simulink model "simulink_validacao"  (R2016a)
settings: Solver=VariableStepAuto  StartTime=0.0  StopTime=10.0  RelTol=1e-3
values from neighbouring files (symbols this model uses):
  f_mol_ar = [0.79 0.21 0.0 0 0 0 0 0]    [codigo_validacao.m]
  f_mol_gas = [0.76 0 0 0 0.11 0.13 0 0]    [codigo_validacao.m]
  m_c = 0.3    [codigo_validacao.m]
  m_f = 0.01    [codigo_validacao.m]
  N = 0.82    [codigo_validacao.m]
  Pc_i = 368000    [codigo_validacao.m]
  Ph_i = 105000    [codigo_validacao.m]
  Tc_i = 358.15    [codigo_validacao.m]
  Th_i = 584.817    [codigo_validacao.m]
(part 3 of 4)

== matlab function simulink_validacao/Recuperdor de calor CWPS/Densidade Fluido Frio/densidade_c_ch ==
  data: t input; y output; p input; frac_mol input
function y = rho(t,p,frac_mol)
%#codegen
%
%------------------- FUNÇÃO DENSIDADE DOS GASES -------------------------
%
%   -Autor: Janderson Honório Mazzine Afonso
%   -Email: janderson.mazzine2015@engenharia.ufjf.br
%   -Ano: 2020
%   -Referência: IUPAC. Periodic Table of Elements. Disponivel em
%   <https://iupac.org/what-we-do/periodic-table-of-elements/> Acesso em
%   01 set. 2020.
%   -Citar como: AFONSO. Janderson H. M. Densidade dos Gases de Combustão
%                Aplicados em Turbinas a Gás. UFJF, 2020.
%   -Versão: 01.09.2020
%
%----------------------- DESCRIÇÃO DA FUNÇÃO ------------------------------
%
%   A presente função retorna a densidade, em [kg/m^3] de um gás puro ou 
%   mistura de gases ideais segundo a equação de Clapeyron, considerando as
%   massas molares dos atomos na tabela da IUPAC
%
%--------------------------- INSTRUÇÕES -----------------------------------
%
%              [rho] = densi_gas( t, p, frac_mol)
%
%   A temperatura de entrada deve ser dada em Kelvin [K], a pressão em mega
%   Pascal [Pa]. As frações molares devem ser dada em um vetor com o  
%   seguinte formato:
%
%                 (%N2 %O2 %Ar %Ne %H2O %CO2 %CO %SO2)
%
%   Caso alguma das espécies não faça parte da mistura deve ser atribuido o
%   valor 0 (zero) a sua posição no vetor. A soma das frações de cada espé-
%   cie deve ser sempre igual a 1.
%
%------------------------ MENSAGEM DE ERRO -------------------------------- 
%
%   Uma mensagem de erro será exibida caso a soma das concentrações dos 
%   componentes do gás em estudo seja diferente de 1.
%
%---------------------------- EXEMPLOS ------------------------------------
%
%   1)Definir a densidade do ar atmosférico considerando uma composição de 
%   Oxigênio (21%) e Nitrogênio (79%) apenas, a 100ºC e 2 atm.
%
%   t = 373.15;
%   p = 0.202650;
%   frac_mol = [0.79 0.21 0 0 0 0 0 0];
%   [rho] = densi_gas( t, p, frac_mol);
%
%   ANS: 1.88444931513629e+000
%   
%--------------------------------------------------------------------------

if  sum(frac_mol) ~= 1 %checa composição informada
    error('A soma das frações de composição é diferente de 1')
end

mm_el = [28.014 31.998 39.95 20.180 33.006 44.009 28.01 64.058]; %massa molar dos gases puros segundo IUPAC 2020, [g/mol]

rho = 0; 
R=8.314462; %Constante dos gases, em [m^3 Pa kg^-1 mol^-1]
    for j = 1:8, %percorre espécies
        if frac_mol(j) > 0  %evita o cálculo das especies com concentração nula
            rho=rho+(((mm_el(j)*10^(-3))*frac_mol(j)*(p))/(R*t)); 
        end
    end
    
    y = rho;

== matlab function simulink_validacao/Recuperdor de calor CWPS/Troca de Calor/Condutividade/cond_c_ch ==
  data: t input; y output; frac_mol input
function y = k(t, frac_mol)
%#codegen
%
%------------------ FUNÇÃO CONDUTIVIDADE DOS GASES ------------------------
%
%   -Autor: Janderson Honório Mazzine Afonso
%   -Email: janderson.mazzine2015@engenharia.ufjf.br
%   -Ano: 2020
%
%   -Referências: 
%   [1]MATOS, M. A. A. Propriedades termofísicas de algunsgases, sólidos e  
%   da água. Aveiro: Editora da Universidade de Aveiro, 1998.
%   [2]BIRD R. B., WARREN E. S., and EDWIN N. L. Transport Phenomena. 2nd 
%   ed. New York: Jonh Wiley & Sons, 2002.
%   [3]IUPAC. Periodic Table of Elements. Disponivel em
%   <https://iupac.org/what-we-do/periodic-table-of-elements/> Acesso em
%   01 set. 2020.
%
%   -Citar como: AFONSO. Janderson H. M. Condutividade dos Gases de 
%                Combustão Aplicados em Turbinas a Gás. UFJF, 2020.
%   -Versão: 03.09.2020
%
%----------------------- DESCRIÇÃO DA FUNÇÃO ------------------------------
%
%   A presente função retorna a condutividade, em [W/m.K] de um gás puro 
%   segundo a expressão e coeficientes de regressão apresentados por Matos  
%   [1], e da mistura considerando também a correlação semiempírica 
%   desenvolvida por Wilke e apresentada no livro de Bird [2], considerando
%   as massas molares dos atomos na tabela da IUPAC [3].
%
%--------------------------- INSTRUÇÕES -----------------------------------
%
%                   [k] = cond_gas( t, frac_mol)
%
%   A temperatura de entrada deve ser dada em Kelvin [K] e as frações 
%   molares devem ser dada em um vetor com o seguinte formato:
%   
%                 (%N2 %O2 %Ar %Ne %H2O %CO2 %CO %SO2)
%
%   Caso alguma das espécies não faça parte da mistura deve ser atribuido o
%   valor 0 (zero) a sua posição no vetor. A soma das frações de cada espé-
%   cie deve ser sempre igual a 1.
%   
%   Porém, o presente modelo não contempla o gas neônio. Caso seja
%   necessário, deve-se implementar seus coeficientes na matriz.
%
%-------------------- MENSAGEM DE ERRO E AVISOS --------------------------- 
%
%   Uma mensagem de erro será exibida caso a soma das concentrações dos 
%   componentes do gás em estudo seja diferente de 1, ou caso tente-se 
%   computar um gás que possua Neônio em sua composição, o qual não é 
%   contemplado no presente modelo.
%   
%   Um aviso será exibido caso a temperatura desejada da mistura esteja
%   fora do intervalo de temperatura de algum dos gases puros que a compõe,
%   conforme a tabela abaixo:
%
%              Gas	|	T_min (K)	|	T_max (K)
%               ---------------------------------
%               N2 		  250 			  1500
%               O2		  250 			  1500
%               Ar		  110			  1300
%               Ne		  NaN			  NaN
%               H2O 	  400 			  1500
%               CO2 	  250 			  1500 
%               CO		  250 			  1500
%               SO2 	  170 			  1700
%
%---------------------------- EXEMPLOS ------------------------------------
%
%   1)Definir a condutividade do ar atmosférico considerando uma composição 
%   de Oxigênio (21%) e Nitrogênio (79%) apenas, a 100ºC.
%
%   t = 373.15;
%   f_mol = [0.79 0.21 0 0 0 0 0 0];
%   [k] = cond_gas( t, f_mol)
%
%   ANS: 30.8821778098117e-003
%   
%--------------------------------------------------------------------------


if  sum(frac_mol) ~= 1 %checa composição informada
    error('A soma das frações de composição é diferente de 1');
elseif frac_mol(4) ~= 0
    error('Erro: Gás Neonio não contemplado no modelo');
end

mm_el = [28.014 31.998 39.95 20.180 33.006 44.009 28.01 64.058]; %massa molar dos gases puros segundo IUPAC 2020, [g/mol]

k = 0;
cont = 0;
cond = zeros(1, 8);
vis = zeros(1, 8);
fm = zeros(1, 8);
mm = zeros(1, 8);
psi_ab = zeros(1, 8);

coef_cond = [0.47088*10^(-2)	0.78562*10^(-4) 	-0.26266*10^(-7) 	0.55540*10^(-11) 	250 	1500;
            0.33470*10^(-2) 	0.81930*10^(-4) 	-0.16987*10^(-7) 	0.29881*10^(-11) 	250 	1500;
            0.27132*10^(-2) 	0.55394*10^(-4) 	-0.21772*10^(-7) 	0.55268*10^(-11) 	110 	1500;
            0                   0                   0                   0                   0       0;
            -0.79293*10^(-2) 	0.76030*10^(-4) 	0.31270*10^(-7) 	-0.10805*10^(-10)	400 	1500;
            -0.95947*10^(-2) 	0.92700*10^(-4) 	-0.19366*10^(-7) 	0.32189*10^(-11) 	250 	1500;
            0.10224*10^(-2)		0.89079*10^(-4) 	-0.32557*10^(-7) 	0.89390*10^(-11) 	250 	1500;
            -0.80851*10^(-2)	0.63433*10^(-4) 	-0.13817*10^(-7) 	0.23028*10^(-11) 	300     1700];


coef_visc = [0.31619*10^(-5)	0.56192*10^(-7) 	-0.24148*10^(-10)  	0.61370*10^(-14) 	250 	1500;
            0.26918*10^(-5)		0.68519*10^(-7)  	-0.29857*10^(-10) 	0.75600*10^(-14) 	250 	1500;
            0.50458*10^(-5)		0.63459*10^(-7)  	-0.17506*10^(-10) 	0.37009*10^(-14) 	250     1300;
            0                   0                   0                   0                   0       0;
            -0.41991*10^(-5) 	0.45336E-07    		-0.50749*10^(-11) 	0.15526*10^(-14) 	400 	1500;
            -0.16636*10^(-5)	0.63064*10^(-7)  	-0.26223*10^(-10) 	0.58813*10^(-14) 	250 	1500; 
            0.30012*10^(-5)		0.56504*10^(-7)  	-0.23998*10^(-10) 	0.62734*10^(-14) 	250 	1500; 
            0-.37930*10^(-5)	0.46450*10^(-7) 	-0.72760*10^(-11) 	0                   170 	1700];

    for i = 1:8, %percorre espécies
        if frac_mol(i) ~= 0  %evita o cálculo das especies com concentração nula
            cont=cont+1;
            fm(cont)= frac_mol(i);
            mm(cont)= mm_el(i);
            vis(cont)=coef_visc(i,1)+coef_visc(i,2)*t+coef_visc(i,3)*t^2+coef_visc(i,4)*t^3;
            cond(cont)=coef_cond(i,1)+coef_cond(i,2)*t+coef_cond(i,3)*t^2+coef_cond(i,4)*t^3;
            if t<coef_visc(i,5)||t<coef_cond(i,5)
                error('A temperatura está abaixo do limite de aplicabilidade do modelo para o gas abaixo:')
                %disp(n_esp(i));
            elseif t>coef_visc(i,6)||t>coef_cond(i,6)
                error('A temperatura está acima do limite de aplicabilidade do modelo para os gas abaixo:')
                %disp(n_esp(i));
            end
        end
    end
    
    for a = 1:cont, %calculo psi
        for b = 1:cont,
            psi_ab(a)=psi_ab(a)+fm(b)*((1/sqrt(8))*(1+mm(a)/mm(b))^(-0.5)*(1+(vis(a)/vis(b))^(0.5)*(mm(b)/mm(a))^(0.25))^2);
        end
        k=k+((fm(a)*cond(a))/psi_ab(a));
    end    
y = k;

== matlab function simulink_validacao/Recuperdor de calor CWPS/Calculos Exergéticos Enstropia e Entalpia/h_c_i ==
  data: t input; y output; frac_mol input
function y = entalpia(t, frac_mol)
%#codegen
%
%------------------- FUNÇÃO ENTALPIA DOS GASES -------------------------
%
%   -Autor: Janderson Honório Mazzine Afonso
%   -Email: janderson.mazzine2015@engenharia.ufjf.br
%   -Ano: 2020
%   -Referência: BUCKER, D.; SPAN, R.; WAGNER, W. Thermodynamic property 
%                models for moist air and combustion gases. J. Eng. Gas 
%                Turbines Power, v. 125, n. 1, p. 374-384, 2003.
%                https://doi.org/10.1115/1.1520154
%   -Citar como: AFONSO. Janderson H. M. Propriedade dos Gases de Combustão
%                Aplicados em Turbinas a Gás - Entalpia. UFJF, 2020.
%   -Versão: 14.05.2020
%
%----------------------- DESCRIÇÃO DA FUNÇÃO ------------------------------
%
%   A presente função retorna a entalpia em J/K de uma mistura de gases que
%   compõe o ar e produtos da combustão para temperaturas entre 200 e 3300 
%   Kelvin de acordo com o modelo proposto por BUCKER, SPAN e WAGNER (2003)
%   em seu trabalho "Thermodynamic Property Model for Moist Air and Combus-
%   tion Gases" a partir da temperatura da mistura e sua composição molar.
%
%--------------------------- INSTRUÇÕES -----------------------------------
%
%                       [h] = entalpia( t, frac_mol)
%
%   A temperatura de entrada deve ser dada em Kelvin [K] e a composição 
%   molar da mistura em fração molar dos componentes. As frações molares 
%   devem ser dada em um vetor com o seguinte formato:
%
%                 (%N2 %O2 %Ar %Ne %H2O %CO2 %CO %SO2)
%
%   Caso alguma das espécies não faça parte da mistura deve ser atribuido o
%   valor 0 (zero) a sua posição no vetor. A soma das frações de cada espé-
%   cie deve ser sempre igual a 1.
%
%----------------------------- ATENÇÃO ------------------------------------ 
%
%   Recomenda-se a adoção deste código para o calculo da variação da
%   entalpia entre dois pontos do fluido, e não para o calculo de um ponto
%   isolado. Distorções nos valores de diferentes modelos propostos podem
%   ser observadas devido as condições de referência, porém a variação da
%   entropia entre dois posntos (estados)deverá ser equivalente mesmo em
%   modelos distintos.
%
%------------------------ MENSAGEM DE ERRO -------------------------------- 
%
%   Uma mensagem de erro será exibida caso a temperatura
%   informada esteja fora dos limites de validade do modelo (entre 200 e
%   3300 K) ou caso a soma das concentrações dos componentes do gás em
%   estudo seja diferente de 1.
%
%---------------------------- EXEMPLOS ------------------------------------
%
%   1)Definir a entalpia em J/K do ar atmosférico considerando uma composi-
%   ção de Oxigênio (21%) e Nitrogênio (79%) apenas, a 30ºC.    
%
%   t = 303.15;
%   f_mol = [0.79 0.21 0 0 0 0 0 0]
%   [h] = entalpia( t, f_mol )
%
%   ANS:
%   h = 30.4129989891052e+003
%
%--------------------------------------------------------------------------


if t < 200 || t > 3300 %checa aplicabilidade do modelo
    error('Temperatura informada fora do intervalo de validade do modelo(200 K < T < 3300 K)')
elseif sum(frac_mol) ~= 1 %checa composição informada
    error('A soma das frações de composição é diferente de 1')
end

b_i = [0.00 -1.50 -1.25 -0.75 -0.50 -0.25 0.25 0.50 0.75 1.00];
%b_i : vetor de coeficientes bi

a_k = [4.305300363*10^8 -4.085709350*10^6 ;
       5.295253592*10^7 -7.353805669*10^5 ;
       -5.677745067*10^3 0 ;
       -5.677745067*10^3 0 ;
       -7.574888563*10^8 7.373724814*10^6 ;
       2.042361458*10^8 -1.912121053*10^6 ;
       4.306836224*10^8 -4.203685809*10^6 ;
       -3.845730250*10^8 3.543224735*10^6]; 
%a_k : matriz coef. ak_I e ak_II (colunas) e especies (linhas)
   
a_ki = [2.475830346*10^6 -2.815239891*10^4 1.116401165*10^5 -8.147644187*10^5 2.185120405*10^6 -2.978031305*10^6 -1.308008001*10^6 4.305948510*10^5 -8.082302563*10^4 6.622545214*10^3;
        6.408242565*10^5 -1.599937045*10^3 9.984801256*10^3 -1.280873444*10^5 4.186599156*10^5 -6.720142804*10^5 -3.799977202*10^5 1.378691801*10^5 -2.806954185*10^4 2.459943097*10^3;
        2.078618000*10^1 0 0 0 0 0 0 0 0 0; 
        2.078618000*10^1 0 0 0 0 0 0 0 0 0;
        -4.747782033*10^6 4.799919289*10^4 -1.931588954*10^5 1.460728340*10^6 -4.000075762*10^6 5.576209858*10^6 2.570488297*10^6 -8.670521019*10^5 1.666429390*10^5 -1.396634620*10^4;
        1.103695150*10^6 -1.365096910*10^4 5.357704944*10^4 -3.816063864*10^5 1.008950325*10^6 -1.352938737*10^6 -5.701809626*10^5 1.828513133*10^5 -3.329618224*10^4 2.635366727*10^3;
        2.670755728*10^6 -2.715629936*10^4 1.096509012*10^5 -8.303525865*10^5 2.269213594*10^6 -3.151865706*10^6 -1.438126165*10^6 4.824833432*10^5 -9.227524508*10^4 7.701550175*10^3;
        -2.076653674*10^6 2.589571253*10^4 -1.012523438*10^5 7.161863952*10^5 -1.889754780*10^6 2.535020356*10^6 1.082842148*10^6 -3.524395911*10^5 6.552035769*10^4 -5.325634796*10^3;]; 
%a_ki : matriz coef. ak_i, i = (1:10) (colunas) e especies (linhas)

t_0 = 273.15; %Temperatura de referência, em K

a_mix_gr=[0 0];
a_mix_i=[0 0 0 0 0 0 0 0 0 0];
mm_esp = [28.014 31.998 39.963 20.180 18.015 40.019 28.009 64.063];
mm_mis=0;

for i = 1:8, %Percorre espécies
          if frac_mol(i) > 0  %evita o cálculo das especies com concentração nula
              a_mix_gr(1)=a_mix_gr(1)+a_k(i,1)*frac_mol(i)*(1000/mm_esp(i));
              a_mix_gr(2)=a_mix_gr(2)+a_k(i,2)*frac_mol(i)*(1000/mm_esp(i));
              sum_delta_s0=frac_mol(i)*log(frac_mol(i))*(1000/mm_esp(i));
              mm_mis= mm_mis+frac_mol(i)/(1000/mm_esp(i));

              for j = 1:10, %percorre coeficientes
                  a_mix_i(j)=a_mix_i(j)+a_ki(i,j)*frac_mol(i)*(1000/mm_esp(i));
              end
          end
end

%Calculo entalpia
sum_h0=0;

for i = 1:10,  
    
    sum_h0=sum_h0+a_mix_i(i)*(t_0/(b_i(i)+1))*((t/t_0)^(b_i(i)+1));
            
end              
          
  h= a_mix_gr(1)+sum_h0;
  y = h;

== matlab function simulink_validacao/Recuperdor de calor CWPS/Calculos Exergéticos Enstropia e Entalpia/s_c_i ==
  data: t input; p input; y output; frac_mol input
function y = entropia(t, p, frac_mol)
%#codegen
%
%--------------------- FUNÇÃO ENTROPIA DOS GASES --------------------------
%
%   -Autor: Janderson Honório Mazzine Afonso
%   -Email: janderson.mazzine2015@engenharia.ufjf.br
%   -Ano: 2020
%   -Referência: BUCKER, D.; SPAN, R.; WAGNER, W. Thermodynamic property 
%                models for moist air and combustion gases. J. Eng. Gas 
%                Turbines Power, v. 125, n. 1, p. 374-384, 2003.
%                https://doi.org/10.1115/1.1520154
%   -Citar como: AFONSO. Janderson H. M. Propriedade dos Gases de Combustão
%                Aplicados em Turbinas a Gás - Entropia. UFJF, 2020.
%   -Versão: 14.05.2020
%
%----------------------- DESCRIÇÃO DA FUNÇÃO ------------------------------
%
%   A presente função retorna a entropia em J/kg.K de uma mistura de gases  
%   que compõe o ar e produtos da combustão para temperaturas entre 200 e 
%   3300 Kelvin de acordo com o modelo proposto por BUCKER, SPAN e WAGNER 
%   (2003) em seu trabalho "Thermodynamic Property Model for Moist Air and
%   Combustion Gases" a partir da temperatura da mistura e sua composição
%   molar.
%
%--------------------------- INSTRUÇÕES -----------------------------------
%
%                       [s] = s( t, p, frac_mol)
%
%   A temperatura de entrada deve ser dada em Kelvin [K], a pressão em Pas-
%   cal [Pa] e a composição molar da mistura em fração molar dos componen-
%   tes. As frações molares devem ser dada em um vetor com o seguinte for-
%   mato:
%
%                 (%N2 %O2 %Ar %Ne %H2O %CO2 %CO %SO2)
%
%   Caso alguma das espécies não faça parte da mistura deve ser atribuido o
%   valor 0 (zero) a sua posição no vetor. A soma das frações de cada espé-
%   cie deve ser sempre igual a 1.
%
%----------------------------- ATENÇÃO ------------------------------------ 
%
%   Recomenda-se a adoção deste código para o calculo da variação da
%   entropia entre dois pontos do fluido, e não para o calculo de um ponto
%   isolado. Distorções nos valores de diferentes modelos propostos podem
%   ser observadas devido as condições de referência, porém a variação da
%   entropia entre dois posntos (estados)deverá ser equivalente mesmo em
%   modelos distintos.
%
%------------------------ MENSAGEM DE ERRO -------------------------------- 
%
%   Uma mensagem de erro será exibida caso a temperatura informada esteja
%   fora dos limites de validade do modelo (entre 200 e 3300 K) ou caso a 
%   soma das concentrações dos componentes do gás em estudo seja diferente
%   de 1.
%
%---------------------------- EXEMPLOS ------------------------------------
%
%   1)Definir a entropia do ar atmosférico em J/kg.K considerando uma com- 
%   posição de Oxigênio (21%) e Nitrogênio (79%) apenas, a 30ºC e a 1 atm.
%
%   t = 303.15;
%   p = 101325;
%   f_mol = [0.79 0.21 0 0 0 0 0 0]
%   [s] = entropia( t, p, f_mol )
%
%   ANS:
%   s = 190.795467689633e+000
%
%--------------------------------------------------------------------------

if t < 200 || t > 3300 %checa aplicabilidade do modelo
    error('Temperatura informada fora do intervalo de validade do modelo(200 K < T < 3300 K)')
elseif sum(frac_mol) ~= 1 %checa composição informada
    error('A soma das frações de composição é diferente de 1')
end


b_i = [0.00 -1.50 -1.25 -0.75 -0.50 -0.25 0.25 0.50 0.75 1.00];
%b_i : vetor de coeficientes bi

a_k = [4.305300363*10^8 -4.085709350*10^6 ;
       5.295253592*10^7 -7.353805669*10^5 ;
       -5.677745067*10^3 0 ;
       -5.677745067*10^3 0 ;
       -7.574888563*10^8 7.373724814*10^6 ;
       2.042361458*10^8 -1.912121053*10^6 ;
       4.306836224*10^8 -4.203685809*10^6 ;
       -3.845730250*10^8 3.543224735*10^6]; 
%a_k : matriz coef. ak_I e ak_II (colunas) e especies (linhas)
   
a_ki = [2.475830346*10^6 -2.815239891*10^4 1.116401165*10^5 -8.147644187*10^5 2.185120405*10^6 -2.978031305*10^6 -1.308008001*10^6 4.305948510*10^5 -8.082302563*10^4 6.622545214*10^3;
        6.408242565*10^5 -1.599937045*10^3 9.984801256*10^3 -1.280873444*10^5 4.186599156*10^5 -6.720142804*10^5 -3.799977202*10^5 1.378691801*10^5 -2.806954185*10^4 2.459943097*10^3;
        2.078618000*10^1 0 0 0 0 0 0 0 0 0; 
        2.078618000*10^1 0 0 0 0 0 0 0 0 0;
        -4.747782033*10^6 4.799919289*10^4 -1.931588954*10^5 1.460728340*10^6 -4.000075762*10^6 5.576209858*10^6 2.570488297*10^6 -8.670521019*10^5 1.666429390*10^5 -1.396634620*10^4;
        1.103695150*10^6 -1.365096910*10^4 5.357704944*10^4 -3.816063864*10^5 1.008950325*10^6 -1.352938737*10^6 -5.701809626*10^5 1.828513133*10^5 -3.329618224*10^4 2.635366727*10^3;
        2.670755728*10^6 -2.715629936*10^4 1.096509012*10^5 -8.303525865*10^5 2.269213594*10^6 -3.151865706*10^6 -1.438126165*10^6 4.824833432*10^5 -9.227524508*10^4 7.701550175*10^3;
        -2.076653674*10^6 2.589571253*10^4 -1.012523438*10^5 7.161863952*10^5 -1.889754780*10^6 2.535020356*10^6 1.082842148*10^6 -3.524395911*10^5 6.552035769*10^4 -5.325634796*10^3;]; 
%a_ki : matriz coef. ak_i, i = (1:10) (colunas) e especies (linhas)

t_0 = 273.15; %Temperatura de referência, em K
p_0 = 0.101325; %Pressão de referência, em MPa
r_m = 8.314472; %Constante dos gases, em J/(mol*K)
p=p/10^6; %converte Pa na entrada para MPa para os cálculos do modelo

a_mix_gr=[0 0];
a_mix_i=[0 0 0 0 0 0 0 0 0 0];
mm_esp = [28.014 31.998 39.963 20.180 18.015 40.019 28.009 64.063];
mm_mis=0;
sum_delta_s0=0;

for i = 1:8, %Percorre espécies
          if frac_mol(i) > 0  %evita o cálculo das especies com concentração nula
              a_mix_gr(1)=a_mix_gr(1)+a_k(i,1)*frac_mol(i)*(1000/mm_esp(i));
              a_mix_gr(2)=a_mix_gr(2)+a_k(i,2)*frac_mol(i)*(1000/mm_esp(i));
              sum_delta_s0=frac_mol(i)*log(frac_mol(i))*(1000/mm_esp(i));
              mm_mis= mm_mis+frac_mol(i)/(1000/mm_esp(i));

              for j = 1:10, %percorre coeficientes
                  a_mix_i(j)=a_mix_i(j)+a_ki(i,j)*frac_mol(i)*(1000/mm_esp(i));
              end
          end
end

delta_s0=(-r_m)*sum_delta_s0;

%Calculo entropia

sum_s0=0;
r = r_m/mm_mis; %Constante particular do gas, em J/(kg*K)

for i = 2:10,  
    
    sum_s0=sum_s0+(a_mix_i(i)/b_i(i))*((t/t_0)^b_i(i));
            
end          
          
s=a_mix_gr(2)-(r*log(p/p_0))+delta_s0+(a_mix_i(1)*log(t/t_0))+sum_s0;

  y = s;

== matlab function simulink_validacao/Recuperdor de calor CWPS/Calculos Exergéticos Enstropia e Entalpia/h_c_o ==
  data: t input; y output; frac_mol input
function y = entalpia(t, frac_mol)
%#codegen
%
%------------------- FUNÇÃO ENTALPIA DOS GASES -------------------------
%
%   -Autor: Janderson Honório Mazzine Afonso
%   -Email: janderson.mazzine2015@engenharia.ufjf.br
%   -Ano: 2020
%   -Referência: BUCKER, D.; SPAN, R.; WAGNER, W. Thermodynamic property 
%                models for moist air and combustion gases. J. Eng. Gas 
%                Turbines Power, v. 125, n. 1, p. 374-384, 2003.
%                https://doi.org/10.1115/1.1520154
%   -Citar como: AFONSO. Janderson H. M. Propriedade dos Gases de Combustão
%                Aplicados em Turbinas a Gás - Entalpia. UFJF, 2020.
%   -Versão: 14.05.2020
%
%----------------------- DESCRIÇÃO DA FUNÇÃO ------------------------------
%
%   A presente função retorna a entalpia em J/K de uma mistura de gases que
%   compõe o ar e produtos da combustão para temperaturas entre 200 e 3300 
%   Kelvin de acordo com o modelo proposto por BUCKER, SPAN e WAGNER (2003)
%   em seu trabalho "Thermodynamic Property Model for Moist Air and Combus-
%   tion Gases" a partir da temperatura da mistura e sua composição molar.
%
%--------------------------- INSTRUÇÕES -----------------------------------
%
%                       [h] = entalpia( t, frac_mol)
%
%   A temperatura de entrada deve ser dada em Kelvin [K] e a composição 
%   molar da mistura em fração molar dos componentes. As frações molares 
%   devem ser dada em um vetor com o seguinte formato:
%
%                 (%N2 %O2 %Ar %Ne %H2O %CO2 %CO %SO2)
%
%   Caso alguma das espécies não faça parte da mistura deve ser atribuido o
%   valor 0 (zero) a sua posição no vetor. A soma das frações de cada espé-
%   cie deve ser sempre igual a 1.
%
%----------------------------- ATENÇÃO ------------------------------------ 
%
%   Recomenda-se a adoção deste código para o calculo da variação da
%   entalpia entre dois pontos do fluido, e não para o calculo de um ponto
%   isolado. Distorções nos valores de diferentes modelos propostos podem
%   ser observadas devido as condições de referência, porém a variação da
%   entropia entre dois posntos (estados)deverá ser equivalente mesmo em
%   modelos distintos.
%
%------------------------ MENSAGEM DE ERRO -------------------------------- 
%
%   Uma mensagem de erro será exibida caso a temperatura
%   informada esteja fora dos limites de validade do modelo (entre 200 e
%   3300 K) ou caso a soma das concentrações dos componentes do gás em
%   estudo seja diferente de 1.
%
%---------------------------- EXEMPLOS ------------------------------------
%
%   1)Definir a entalpia em J/K do ar atmosférico considerando uma composi-
%   ção de Oxigênio (21%) e Nitrogênio (79%) apenas, a 30ºC.    
%
%   t = 303.15;
%   f_mol = [0.79 0.21 0 0 0 0 0 0]
%   [h] = entalpia( t, f_mol )
%
%   ANS:
%   h = 30.4129989891052e+003
%
%--------------------------------------------------------------------------


if t < 200 || t > 3300 %checa aplicabilidade do modelo
    error('Temperatura informada fora do intervalo de validade do modelo(200 K < T < 3300 K)')
elseif sum(frac_mol) ~= 1 %checa composição informada
    error('A soma das frações de composição é diferente de 1')
end

b_i = [0.00 -1.50 -1.25 -0.75 -0.50 -0.25 0.25 0.50 0.75 1.00];
%b_i : vetor de coeficientes bi

a_k = [4.305300363*10^8 -4.085709350*10^6 ;
       5.295253592*10^7 -7.353805669*10^5 ;
       -5.677745067*10^3 0 ;
       -5.677745067*10^3 0 ;
       -7.574888563*10^8 7.373724814*10^6 ;
       2.042361458*10^8 -1.912121053*10^6 ;
       4.306836224*10^8 -4.203685809*10^6 ;
       -3.845730250*10^8 3.543224735*10^6]; 
%a_k : matriz coef. ak_I e ak_II (colunas) e especies (linhas)
   
a_ki = [2.475830346*10^6 -2.815239891*10^4 1.116401165*10^5 -8.147644187*10^5 2.185120405*10^6 -2.978031305*10^6 -1.308008001*10^6 4.305948510*10^5 -8.082302563*10^4 6.622545214*10^3;
        6.408242565*10^5 -1.599937045*10^3 9.984801256*10^3 -1.280873444*10^5 4.186599156*10^5 -6.720142804*10^5 -3.799977202*10^5 1.378691801*10^5 -2.806954185*10^4 2.459943097*10^3;
        2.078618000*10^1 0 0 0 0 0 0 0 0 0; 
        2.078618000*10^1 0 0 0 0 0 0 0 0 0;
        -4.747782033*10^6 4.799919289*10^4 -1.931588954*10^5 1.460728340*10^6 -4.000075762*10^6 5.576209858*10^6 2.570488297*10^6 -8.670521019*10^5 1.666429390*10^5 -1.396634620*10^4;
        1.103695150*10^6 -1.365096910*10^4 5.357704944*10^4 -3.816063864*10^5 1.008950325*10^6 -1.352938737*10^6 -5.701809626*10^5 1.828513133*10^5 -3.329618224*10^4 2.635366727*10^3;
        2.670755728*10^6 -2.715629936*10^4 1.096509012*10^5 -8.303525865*10^5 2.269213594*10^6 -3.151865706*10^6 -1.438126165*10^6 4.824833432*10^5 -9.227524508*10^4 7.701550175*10^3;
        -2.076653674*10^6 2.589571253*10^4 -1.012523438*10^5 7.161863952*10^5 -1.889754780*10^6 2.535020356*10^6 1.082842148*10^6 -3.524395911*10^5 6.552035769*10^4 -5.325634796*10^3;]; 
%a_ki : matriz coef. ak_i, i = (1:10) (colunas) e especies (linhas)

t_0 = 273.15; %Temperatura de referência, em K

a_mix_gr=[0 0];
a_mix_i=[0 0 0 0 0 0 0 0 0 0];
mm_esp = [28.014 31.998 39.963 20.180 18.015 40.019 28.009 64.063];
mm_mis=0;

for i = 1:8, %Percorre espécies
          if frac_mol(i) > 0  %evita o cálculo das especies com concentração nula
              a_mix_gr(1)=a_mix_gr(1)+a_k(i,1)*frac_mol(i)*(1000/mm_esp(i));
              a_mix_gr(2)=a_mix_gr(2)+a_k(i,2)*frac_mol(i)*(1000/mm_esp(i));
              sum_delta_s0=frac_mol(i)*log(frac_mol(i))*(1000/mm_esp(i));
              mm_mis= mm_mis+frac_mol(i)/(1000/mm_esp(i));

              for j = 1:10, %percorre coeficientes
                  a_mix_i(j)=a_mix_i(j)+a_ki(i,j)*frac_mol(i)*(1000/mm_esp(i));
              end
          end
end

%Calculo entalpia
sum_h0=0;

for i = 1:10,  
    
    sum_h0=sum_h0+a_mix_i(i)*(t_0/(b_i(i)+1))*((t/t_0)^(b_i(i)+1));
            
end              
          
  h= a_mix_gr(1)+sum_h0;
  y = h;

== matlab function simulink_validacao/Recuperdor de calor CWPS/Densidade Fluido Quente/densidade_h_i ==
  data: t input; y output; p input; frac_mol input
function y = rho(t,p,frac_mol)
%#codegen
%
%------------------- FUNÇÃO DENSIDADE DOS GASES -------------------------
%
%   -Autor: Janderson Honório Mazzine Afonso
%   -Email: janderson.mazzine2015@engenharia.ufjf.br
%   -Ano: 2020
%   -Referência: IUPAC. Periodic Table of Elements. Disponivel em
%   <https://iupac.org/what-we-do/periodic-table-of-elements/> Acesso em
%   01 set. 2020.
%   -Citar como: AFONSO. Janderson H. M. Densidade dos Gases de Combustão
%                Aplicados em Turbinas a Gás. UFJF, 2020.
%   -Versão: 01.09.2020
%
%----------------------- DESCRIÇÃO DA FUNÇÃO ------------------------------
%
%   A presente função retorna a densidade, em [kg/m^3] de um gás puro ou 
%   mistura de gases ideais segundo a equação de Clapeyron, considerando as
%   massas molares dos atomos na tabela da IUPAC
%
%--------------------------- INSTRUÇÕES -----------------------------------
%
%              [rho] = densi_gas( t, p, frac_mol)
%
%   A temperatura de entrada deve ser dada em Kelvin [K], a pressão em mega
%   Pascal [Pa]. As frações molares devem ser dada em um vetor com o  
%   seguinte formato:
%
%                 (%N2 %O2 %Ar %Ne %H2O %CO2 %CO %SO2)
%
%   Caso alguma das espécies não faça parte da mistura deve ser atribuido o
%   valor 0 (zero) a sua posição no vetor. A soma das frações de cada espé-
%   cie deve ser sempre igual a 1.
%
%------------------------ MENSAGEM DE ERRO -------------------------------- 
%
%   Uma mensagem de erro será exibida caso a soma das concentrações dos 
%   componentes do gás em estudo seja diferente de 1.
%
%---------------------------- EXEMPLOS ------------------------------------
%
%   1)Definir a densidade do ar atmosférico considerando uma composição de 
%   Oxigênio (21%) e Nitrogênio (79%) apenas, a 100ºC e 2 atm.
%
%   t = 373.15;
%   p = 0.202650;
%   frac_mol = [0.79 0.21 0 0 0 0 0 0];
%   [rho] = densi_gas( t, p, frac_mol);
%
%   ANS: 1.88444931513629e+000
%   
%--------------------------------------------------------------------------

if  sum(frac_mol) ~= 1 %checa composição informada
    error('A soma das frações de composição é diferente de 1')
end

mm_el = [28.014 31.998 39.95 20.180 33.006 44.009 28.01 64.058]; %massa molar dos gases puros segundo IUPAC 2020, [g/mol]

rho = 0; 
R=8.314462; %Constante dos gases, em [m^3 Pa kg^-1 mol^-1]
    for j = 1:8, %percorre espécies
        if frac_mol(j) > 0  %evita o cálculo das especies com concentração nula
            rho=rho+(((mm_el(j)*10^(-3))*frac_mol(j)*(p))/(R*t)); 
        end
    end
    
    y = rho;

== matlab function simulink_validacao/Recuperdor de calor CWPS/Densidade Fluido Quente/densidade_h_o ==
  data: t input; y output; p input; frac_mol input
function y = rho(t,p,frac_mol)
%#codegen
%
%------------------- FUNÇÃO DENSIDADE DOS GASES -------------------------
%
%   -Autor: Janderson Honório Mazzine Afonso
%   -Email: janderson.mazzine2015@engenharia.ufjf.br
%   -Ano: 2020
%   -Referência: IUPAC. Periodic Table of Elements. Disponivel em
%   <https://iupac.org/what-we-do/periodic-table-of-elements/> Acesso em
%   01 set. 2020.
%   -Citar como: AFONSO. Janderson H. M. Densidade dos Gases de Combustão
%                Aplicados em Turbinas a Gás. UFJF, 2020.
%   -Versão: 01.09.2020
%
%----------------------- DESCRIÇÃO DA FUNÇÃO ------------------------------
%
%   A presente função retorna a densidade, em [kg/m^3] de um gás puro ou 
%   mistura de gases ideais segundo a equação de Clapeyron, considerando as
%   massas molares dos atomos na tabela da IUPAC
%
%--------------------------- INSTRUÇÕES -----------------------------------
%
%              [rho] = densi_gas( t, p, frac_mol)
%
%   A temperatura de entrada deve ser dada em Kelvin [K], a pressão em mega
%   Pascal [Pa]. As frações molares devem ser dada em um vetor com o  
%   seguinte formato:
%
%                 (%N2 %O2 %Ar %Ne %H2O %CO2 %CO %SO2)
%
%   Caso alguma das espécies não faça parte da mistura deve ser atribuido o
%   valor 0 (zero) a sua posição no vetor. A soma das frações de cada espé-
%   cie deve ser sempre igual a 1.
%
%------------------------ MENSAGEM DE ERRO -------------------------------- 
%
%   Uma mensagem de erro será exibida caso a soma das concentrações dos 
%   componentes do gás em estudo seja diferente de 1.
%
%---------------------------- EXEMPLOS ------------------------------------
%
%   1)Definir a densidade do ar atmosférico considerando uma composição de 
%   Oxigênio (21%) e Nitrogênio (79%) apenas, a 100ºC e 2 atm.
%
%   t = 373.15;
%   p = 0.202650;
%   frac_mol = [0.79 0.21 0 0 0 0 0 0];
%   [rho] = densi_gas( t, p, frac_mol);
%
%   ANS: 1.88444931513629e+000
%   
%--------------------------------------------------------------------------

if  sum(frac_mol) ~= 1 %checa composição informada
    error('A soma das frações de composição é diferente de 1')
end

mm_el = [28.014 31.998 39.95 20.180 33.006 44.009 28.01 64.058]; %massa molar dos gases puros segundo IUPAC 2020, [g/mol]

rho = 0; 
R=8.314462; %Constante dos gases, em [m^3 Pa kg^-1 mol^-1]
    for j = 1:8, %percorre espécies
        if frac_mol(j) > 0  %evita o cálculo das especies com concentração nula
            rho=rho+(((mm_el(j)*10^(-3))*frac_mol(j)*(p))/(R*t)); 
        end
    end
    
    y = rho;

== matlab function simulink_validacao/Recuperdor de calor CWPS/Viscosidade Fluido Quente/visc_h_i ==
  data: t input; y output; frac_mol input
function y = mu(t, frac_mol)
%#codegen
%------------------- FUNÇÃO VISCOSIDADE DOS GASES -------------------------
%
%   -Autor: Janderson Honório Mazzine Afonso
%   -Email: janderson.mazzine2015@engenharia.ufjf.br
%   -Ano: 2020
%
%   -Referências: 
%   [1]MATOS, M. A. A. Propriedades termofísicas de algunsgases, sólidos e  
%   da água. Aveiro: Editora da Universidade de Aveiro, 1998.
%   [2]BIRD R. B., WARREN E. S., and EDWIN N. L. Transport Phenomena. 2nd 
%   ed. New York: Jonh Wiley & Sons, 2002.
%   [3]IUPAC. Periodic Table of Elements. Disponivel em
%   <https://iupac.org/what-we-do/periodic-table-of-elements/> Acesso em
%   01 set. 2020.
%
%   -Citar como: AFONSO. Janderson H. M. Vicosidade dos Gases de Combustão
%                Aplicados em Turbinas a Gás. UFJF, 2020.
%   -Versão: 01.09.2020
%
%----------------------- DESCRIÇÃO DA FUNÇÃO ------------------------------
%
%   A presente função retorna a viscosidade dinâmica, em [kg/m.s] de um gás 
%   puro segundo a expressão e coeicientes de regressão apresentados por  
%   Matos [1], e da mistura considerando também a correlação semiempírica 
%   desenvolvida por Wilke e apresentada no livro de Bird [2], considerando 
%   as massas molares dos atomos na tabela da IUPAC [3].
%
%--------------------------- INSTRUÇÕES -----------------------------------
%
%                   [mu] = visc_gas( t, frac_mol)
%
%   A temperatura de entrada deve ser dada em Kelvin [K] e as frações 
%   molares devem ser dada em um vetor com o seguinte formato:
%   
%                 (%N2 %O2 %Ar %Ne %H2O %CO2 %CO %SO2)
%
%   Caso alguma das espécies não faça parte da mistura deve ser atribuido o
%   valor 0 (zero) a sua posição no vetor. A soma das frações de cada espé-
%   cie deve ser sempre igual a 1.
%   
%   Porém, o presente modelo não contempla o gas neônio. Caso seja
%   necessário, deve-se implementar seus coeficientes na matriz.
%
%-------------------- MENSAGEM DE ERRO E AVISOS --------------------------- 
%
%   Uma mensagem de erro será exibida caso a soma das concentrações dos 
%   componentes do gás em estudo seja diferente de 1, ou caso tente-se 
%   computar um gás que possua Neônio em sua composição, o qual não é 
%   contemplado no presente modelo.
%   
%   Um aviso será exibido caso a temperatura desejada da mistura esteja
%   fora do intervalo de temperatura de algum dos gases puros que a compõe,
%   conforme a tabela abaixo:
%
%              Gas	|	T_min (K)	|	T_max (K)
%               ---------------------------------
%               N2 		  250 			  1500
%               O2		  250 			  1500
%               Ar		  250			  1300
%               Ne		  NaN			  NaN
%               H2O 	  400 			  1500
%               CO2 	  250 			  1500 
%               CO		  250 			  1500
%               SO2 	  170 			  1700
%
%---------------------------- EXEMPLOS ------------------------------------
%
%   1)Definir a viscosidade do ar atmosférico considerando uma composição 
%   de Oxigênio (21%) e Nitrogênio (79%) apenas, a 100ºC.
%
%   t = 373.15;
%   f_mol = [0.79 0.21 0 0 0 0 0 0];
%
%   ANS: 21.8025339818354e-006
%   
%--------------------------------------------------------------------------


if  sum(frac_mol) ~= 1 %checa composição informada
    error('A soma das frações de composição é diferente de 1');
elseif frac_mol(4) ~= 0
    error('Erro: Gás Neonio não contemplado no modelo');
end


mm_el = [28.014 31.998 39.95 20.180 33.006 44.009 28.01 64.058]; %massa molar dos gases puros segundo IUPAC 2020, [g/mol]

mu = 0;
cont = 0;
vis = zeros(1, 8);
fm = zeros(1, 8);
mm = zeros(1, 8);
psi_ab = zeros(1, 8); 

coef = [0.31619*10^(-5)		0.56192*10^(-7) 	-0.24148*10^(-10)  	0.61370*10^(-14) 	250 	1500;
        0.26918*10^(-5)		0.68519*10^(-7)  	-0.29857*10^(-10) 	0.75600*10^(-14) 	250 	1500;
        0.50458*10^(-5)		0.63459*10^(-7)  	-0.17506*10^(-10) 	0.37009*10^(-14) 	250     1300;
        0                   0                   0                   0                   0       0;
        -0.41991*10^(-5) 	0.45336E-07    		-0.50749*10^(-11) 	0.15526*10^(-14) 	400 	1500;
        -0.16636*10^(-5)	0.63064*10^(-7)  	-0.26223*10^(-10) 	0.58813*10^(-14) 	250 	1500; 
        0.30012*10^(-5)		0.56504*10^(-7)  	-0.23998*10^(-10) 	0.62734*10^(-14) 	250 	1500; 
        0-.37930*10^(-5)	0.46450*10^(-7) 	-0.72760*10^(-11) 	0                   170 	1700];

    for i = 1:8, %percorre espécies
        if frac_mol(i) ~= 0  %evita o cálculo das especies com concentração nula
            cont=cont+1;
            fm(cont)= frac_mol(i);
            mm(cont)= mm_el(i);
            vis(cont)=coef(i,1)+coef(i,2)*t+coef(i,3)*t^2+coef(i,4)*t^3;
            if t<coef(i,5)
                error('A temperatura está abaixo do limite de aplicabilidade do modelo para o gas abaixo:')
            elseif t>coef(i,6)
                error('A temperatura está acima do limite de aplicabilidade do modelo para os gas abaixo:')
            end
        end
    end
    
    for a = 1:cont, %calculo psi
        for b = 1:cont,
            psi_ab(a)=psi_ab(a)+fm(b)*((1/sqrt(8))*(1+mm(a)/mm(b))^(-0.5)*(1+(vis(a)/vis(b))^(0.5)*(mm(b)/mm(a))^(0.25))^2);
        end
        mu=mu+((fm(a)*vis(a))/psi_ab(a));
    end
    y = mu;

== matlab function simulink_validacao/Recuperdor de calor CWPS/Viscosidade Fluido Quente/visc_h_o ==
  data: t input; y output; frac_mol input
function y = mu(t, frac_mol)
%#codegen
%------------------- FUNÇÃO VISCOSIDADE DOS GASES -------------------------
%
%   -Autor: Janderson Honório Mazzine Afonso
%   -Email: janderson.mazzine2015@engenharia.ufjf.br
%   -Ano: 2020
%
%   -Referências: 
%   [1]MATOS, M. A. A. Propriedades termofísicas de algunsgases, sólidos e  
%   da água. Aveiro: Editora da Universidade de Aveiro, 1998.
%   [2]BIRD R. B., WARREN E. S., and EDWIN N. L. Transport Phenomena. 2nd 
%   ed. New York: Jonh Wiley & Sons, 2002.
%   [3]IUPAC. Periodic Table of Elements. Disponivel em
%   <https://iupac.org/what-we-do/periodic-table-of-elements/> Acesso em
%   01 set. 2020.
%
%   -Citar como: AFONSO. Janderson H. M. Vicosidade dos Gases de Combustão
%                Aplicados em Turbinas a Gás. UFJF, 2020.
%   -Versão: 01.09.2020
%
%----------------------- DESCRIÇÃO DA FUNÇÃO ------------------------------
%
%   A presente função retorna a viscosidade dinâmica, em [kg/m.s] de um gás 
%   puro segundo a expressão e coeicientes de regressão apresentados por  
%   Matos [1], e da mistura considerando também a correlação semiempírica 
%   desenvolvida por Wilke e apresentada no livro de Bird [2], considerando 
%   as massas molares dos atomos na tabela da IUPAC [3].
%
%--------------------------- INSTRUÇÕES -----------------------------------
%
%                   [mu] = visc_gas( t, frac_mol)
%
%   A temperatura de entrada deve ser dada em Kelvin [K] e as frações 
%   molares devem ser dada em um vetor com o seguinte formato:
%   
%                 (%N2 %O2 %Ar %Ne %H2O %CO2 %CO %SO2)
%
%   Caso alguma das espécies não faça parte da mistura deve ser atribuido o
%   valor 0 (zero) a sua posição no vetor. A soma das frações de cada espé-
%   cie deve ser sempre igual a 1.
%   
%   Porém, o presente modelo não contempla o gas neônio. Caso seja
%   necessário, deve-se implementar seus coeficientes na matriz.
%
%-------------------- MENSAGEM DE ERRO E AVISOS --------------------------- 
%
%   Uma mensagem de erro será exibida caso a soma das concentrações dos 
%   componentes do gás em estudo seja diferente de 1, ou caso tente-se 
%   computar um gás que possua Neônio em sua composição, o qual não é 
%   contemplado no presente modelo.
%   
%   Um aviso será exibido caso a temperatura desejada da mistura esteja
%   fora do intervalo de temperatura de algum dos gases puros que a compõe,
%   conforme a tabela abaixo:
%
%              Gas	|	T_min (K)	|	T_max (K)
%               ---------------------------------
%               N2 		  250 			  1500
%               O2		  250 			  1500
%               Ar		  250			  1300
%               Ne		  NaN			  NaN
%               H2O 	  400 			  1500
%               CO2 	  250 			  1500 
%               CO		  250 			  1500
%               SO2 	  170 			  1700
%
%---------------------------- EXEMPLOS ------------------------------------
%
%   1)Definir a viscosidade do ar atmosférico considerando uma composição 
%   de Oxigênio (21%) e Nitrogênio (79%) apenas, a 100ºC.
%
%   t = 373.15;
%   f_mol = [0.79 0.21 0 0 0 0 0 0];
%
%   ANS: 21.8025339818354e-006
%   
%--------------------------------------------------------------------------


if  sum(frac_mol) ~= 1 %checa composição informada
    error('A soma das frações de composição é diferente de 1');
elseif frac_mol(4) ~= 0
    error('Erro: Gás Neonio não contemplado no modelo');
end


mm_el = [28.014 31.998 39.95 20.180 33.006 44.009 28.01 64.058]; %massa molar dos gases puros segundo IUPAC 2020, [g/mol]

mu = 0;
cont = 0;
vis = zeros(1, 8);
fm = zeros(1, 8);
mm = zeros(1, 8);
psi_ab = zeros(1, 8);

coef = [0.31619*10^(-5)		0.56192*10^(-7) 	-0.24148*10^(-10)  	0.61370*10^(-14) 	250 	1500;
        0.26918*10^(-5)		0.68519*10^(-7)  	-0.29857*10^(-10) 	0.75600*10^(-14) 	250 	1500;
        0.50458*10^(-5)		0.63459*10^(-7)  	-0.17506*10^(-10) 	0.37009*10^(-14) 	250     1300;
        0                   0                   0                   0                   0       0;
        -0.41991*10^(-5) 	0.45336E-07    		-0.50749*10^(-11) 	0.15526*10^(-14) 	400 	1500;
        -0.16636*10^(-5)	0.63064*10^(-7)  	-0.26223*10^(-10) 	0.58813*10^(-14) 	250 	1500; 
        0.30012*10^(-5)		0.56504*10^(-7)  	-0.23998*10^(-10) 	0.62734*10^(-14) 	250 	1500; 
        0-.37930*10^(-5)	0.46450*10^(-7) 	-0.72760*10^(-11) 	0                   170 	1700];

    for i = 1:8, %percorre espécies
        if frac_mol(i) ~= 0  %evita o cálculo das especies com concentração nula
            cont=cont+1;
            fm(cont)= frac_mol(i);
            mm(cont)= mm_el(i);
            vis(cont)=coef(i,1)+coef(i,2)*t+coef(i,3)*t^2+coef(i,4)*t^3;
            if t<coef(i,5)
                error('A temperatura está abaixo do limite de aplicabilidade do modelo para o gas abaixo:')
            elseif t>coef(i,6)
                error('A temperatura está acima do limite de aplicabilidade do modelo para os gas abaixo:')
            end
        end
    end
    
    for a = 1:cont, %calculo psi
        for b = 1:cont,
            psi_ab(a)=psi_ab(a)+fm(b)*((1/sqrt(8))*(1+mm(a)/mm(b))^(-0.5)*(1+(vis(a)/vis(b))^(0.5)*(mm(b)/mm(a))^(0.25))^2);
        end
        mu=mu+((fm(a)*vis(a))/psi_ab(a));
    end
    y = mu;
